simulink model "publish_setpoint_raw"  (R2021a)
settings: Solver=FixedStepAuto  StartTime=0.0  StopTime=100  FixedStep=0.004  RelTol=1e-3
InitFcn:
  | rosshutdown
  | rosinit
values from neighbouring files (symbols this model uses):
  Ts_pos_control = 0.01    [initialise_ros_iris_payload.m]
undefined symbols (not defined in the file or in its folder): Position, TypeMask, Yaw
libraries: robotlib x5, robotgazebolib x1
settings Model: SimulationMode=accelerator  Creator=esl  LastModifiedBy=esl
settings OptimizationCC: EnhancedBackFolding=on  PassReuseOutputArgsAs=Individual arguments  ZeroExternalMemoryAtStartup=off  ZeroInternalMemoryAtStartup=off  MaxStackSize=64  OptimizeBlockOrder=speed  DifferentSizesBufferReuse=on  OptimizationCustomize=off  EfficientTunableParamExpr=on
settings DebuggingCC: ParameterTunabilityLossMsg=error
settings HardwareCC: ProdBitPerLong=64  ProdHWDeviceType=Intel->x86-64 (Linux 64)  UseEmbeddedCoderFeatures=off
settings SFSimCC: MATLABDynamicMemAlloc=off
settings RTWCC: SystemTargetFile=ert.tlc  HardwareBoard=Robot Operating System (ROS)  TLCOptions="-aInlineSetEventsForThisBaseRateFcn=TLC_FALSE -aSuppressMultiTaskScheduler=TLC_FALSE  -aRateBasedStepFcn=0"  TemplateMakefile=ert_default_tmf  Toolchain=Catkin  TargetLang=C++
settings CodeAppCC: ForceParamTrailComments=on  IgnoreCustomStorageClasses=off  OperatorAnnotations=on  SimulinkDataObjDesc=on  SFDataObjDesc=on  InsertBlockDesc=on
settings ERTTargetCC: SupportNonInlinedSFcns=on

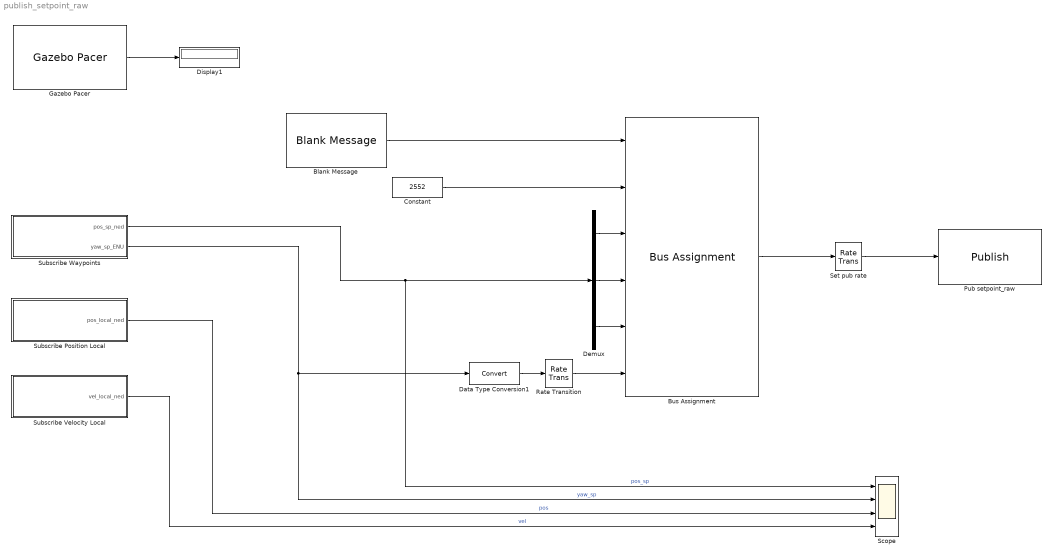
== system publish_setpoint_raw ==
  Blank Message : robotlib/Blank Message  messageClass=Message  entityType=mavros_msgs/PositionTarget  messageType=mavros_msgs/PositionTarget  SampleTime=inf  legacyBusStruct=off
  Bus Assignment : BusAssignment  AssignedSignals=TypeMask,Position.X,Position.Y,Position.Z,Yaw
  Constant : Constant  Value=2552  OutDataTypeStr=Inherit: Inherit via back propagation
  Data Type Conversion1 : DataTypeConversion
  Demux : Demux  Outputs=3
  Display1 : Display
  Gazebo Pacer : robotgazebolib/Gazebo Pacer  ResetBehavior=Reset Gazebo simulation time  SampleTime=0.004
      settings: SourceProductBaseCode=RO
  Pub setpoint_raw : robotlib/Publish  topicSource=Select from ROS network  topic=/mavros/setpoint_raw/local  messageType=mavros_msgs/PositionTarget  legacyBusStruct=off  messageQueueLength=1
  Rate Transition : RateTransition  OutPortSampleTimeOpt=Inherit  OutPortSampleTime=0.03
  Scope : Scope  NumInputPorts=4
  Set pub rate : RateTransition  OutPortSampleTime=Ts_pub_setpoint
  Subscribe Position Local : Subsystem
  Subscribe Velocity Local : Subsystem
  Subscribe Waypoints : Subsystem
  wires:
  Subscribe Waypoints/1(pos_sp_ned) -> Scope/1, Demux/1  "pos_sp"
  Gazebo Pacer/1 -> Display1/1
  Set pub rate/1 -> Pub setpoint_raw/1
  Constant/1 -> Bus Assignment/2
  Blank Message/1 -> Bus Assignment/1
  Data Type Conversion1/1 -> Rate Transition/1
  Rate Transition/1 -> Bus Assignment/6
  Bus Assignment/1 -> Set pub rate/1
  Subscribe Waypoints/2(yaw_sp_ENU) -> Scope/2, Data Type Conversion1/1  "yaw_sp"
  Demux/2 -> Bus Assignment/4
  Demux/1 -> Bus Assignment/3
  Demux/3 -> Bus Assignment/5
  Subscribe Position Local/1(pos_local_ned) -> Scope/3  "pos"
  Subscribe Velocity Local/1(vel_local_ned) -> Scope/4  "vel"

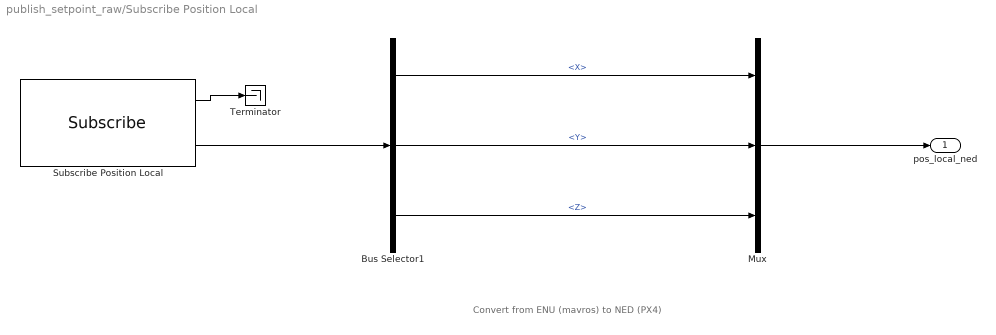
== system publish_setpoint_raw/Subscribe Position Local ==
  note: Convert from ENU (mavros) to NED (PX4)
  Bus Selector1 : BusSelector  OutputSignals=Pose.Position.X,Pose.Position.Y,Pose.Position.Z
  Mux : Mux  Inputs=3
  Subscribe Position Local : robotlib/Subscribe  topicSource=Select from ROS network  topic=/mavros/local_position/pose  messageType=geometry_msgs/PoseStamped  SampleTime=Ts_pos_control  legacyBusStruct=off  messageQueueLength=1
  Terminator : Terminator
  pos_local_ned : Outport
  wires:
  Subscribe Position Local/1 -> Terminator/1
  Mux/1 -> pos_local_ned/1
  Subscribe Position Local/2 -> Bus Selector1/1
  Bus Selector1/1 -> Mux/1  "<X>"
  Bus Selector1/2 -> Mux/2  "<Y>"
  Bus Selector1/3 -> Mux/3  "<Z>"

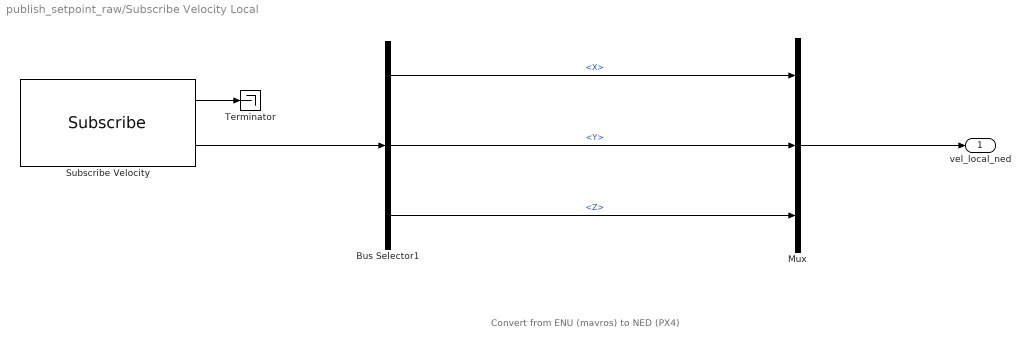
== system publish_setpoint_raw/Subscribe Velocity Local ==
  note: Convert from ENU (mavros) to NED (PX4)
  Bus Selector1 : BusSelector  OutputSignals=Twist.Linear.X,Twist.Linear.Y,Twist.Linear.Z
  Mux : Mux  Inputs=3
  Subscribe Velocity : robotlib/Subscribe  topicSource=Select from ROS network  topic=/mavros/local_position/velocity_local  messageType=geometry_msgs/TwistStamped  SampleTime=Ts_pos_control  legacyBusStruct=off  messageQueueLength=1
  Terminator : Terminator
  vel_local_ned : Outport
  wires:
  Subscribe Velocity/1 -> Terminator/1
  Subscribe Velocity/2 -> Bus Selector1/1
  Mux/1 -> vel_local_ned/1
  Bus Selector1/1 -> Mux/1  "<X>"
  Bus Selector1/2 -> Mux/2  "<Y>"
  Bus Selector1/3 -> Mux/3  "<Z>"

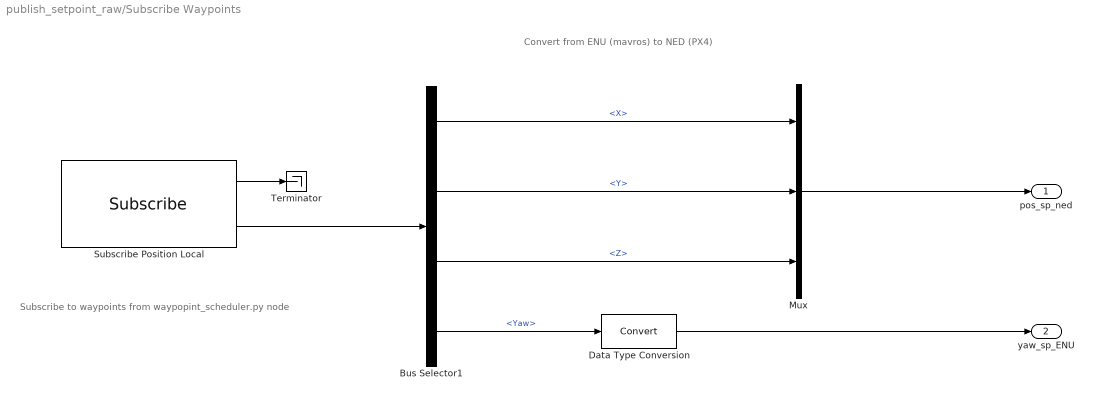
== system publish_setpoint_raw/Subscribe Waypoints ==
  note: Subscribe to waypoints from waypopint_scheduler.py node
  note: Convert from ENU (mavros) to NED (PX4)
  Bus Selector1 : BusSelector  OutputSignals=Position.X,Position.Y,Position.Z,Yaw
  Data Type Conversion : DataTypeConversion
  Mux : Mux  Inputs=3
  Subscribe Position Local : robotlib/Subscribe  topicSource=Select from ROS network  topic=/setpoint_raw/local  messageType=mavros_msgs/PositionTarget  SampleTime=Ts_pos_control  legacyBusStruct=off  messageQueueLength=1
  Terminator : Terminator
  pos_sp_ned : Outport
  yaw_sp_ENU : Outport  Port=2
  wires:
  Subscribe Position Local/1 -> Terminator/1
  Subscribe Position Local/2 -> Bus Selector1/1
  Bus Selector1/1 -> Mux/1  "<X>"
  Bus Selector1/2 -> Mux/2  "<Y>"
  Bus Selector1/3 -> Mux/3  "<Z>"
  Bus Selector1/4 -> Data Type Conversion/1  "<Yaw>"
  Mux/1 -> pos_sp_ned/1
  Data Type Conversion/1 -> yaw_sp_ENU/1
